simulink model "hdv_hydroelectropowertrain_model"  (R2023b)
settings: Solver=ode1be  StartTime=0.0  StopTime=simulation_length  FixedStep=tsample  MaxStep=tsample
values from neighbouring files (symbols this model uses):
  alpha = 35    [init_model.m]
  Apump = [0 1; 0 0]    [init_model.m]
  available_torque = torque_base+torque_friction_base    [init_model.m]
  Bpump = [0 1]'    [init_model.m]
  btheta_shaft = 2e2    (= 200)    [init_model.m]
  C1 = 10    [init_model.m]
  consumption = [consumption_1, consumption_2, consumption_3, consumption_4,          consumption_5, consumption_6, consumption_7, consumption_8,          consumption_9, consumption_10, consumption_11, consumption_12,          consumption_13, consumption_14, consumption_15, consumption_16          ]    [ic_engine_data.m]
  Cpump = [k 0]    [init_model.m]
  dp_lim = 400    [init_model.m]
  E0 = 3.685    [init_model.m]
  E1 = 0.2156    [init_model.m]
  E2 = 0    [init_model.m]
  E3 = 0    [init_model.m]
  E_1 = -1.031    [init_model.m]
  Elog = -0.05    [init_model.m]
  eta_v_m = 0.98    [init_model.m]
  eta_v_p = 0.97    [init_model.m]
  ki_dp_comp = 1/dp_lim    (= 0.0025)    [init_model.m]
  ki_te_comp = 2/te_lim    [init_model.m]
  kp_ctrl_m = 1    [init_model.m]
  kp_dp_comp = 0.5/dp_lim    (= 0.00125)    [init_model.m]
  kp_te_comp = 1/te_lim    [init_model.m]
  Kpump = acker(Apump,Bpump,poles)    [init_model.m]
  load_blade_enable = 0    [init_model.m]
  Lpump = acker(Apump',Cpump',pole_so)'    [init_model.m]
  M = 125    [init_model.m]
  Ncell = 185    [init_model.m]
  Npump = -1/(Cpump*inv(Apump-Bpump*Kpump)*Bpump)    [init_model.m]
  omega_e_rpm_ref = 1700    [init_model.m]
  omega_l_max_rpm = omega_l_max/(2*pi)*60    (= 50.3075969543)    [init_model.m]
  q1Kalman = tsample^2*1e-2    (= 1e-08)    [init_model.m]
  q2Kalman = tsample^1*1e-1    (= 0.0001)    [init_model.m]
  q3Kalman = 0    [init_model.m]
  Qhr = 400    [init_model.m]
  R0 = 0.015    [init_model.m]
  R1 = 0.015    [init_model.m]
  R_tg = 1.16/2    (= 0.58)    [init_model.m]
  rKalman = 1    [init_model.m]
  rpm_base = [620 700 800 900 1000 1100 1200 1300 1400 1500 1600 1700 1800      1900 2000 2100]    [ic_engine_data.m]
  rpm_consumption = rpm_base    [ic_engine_data.m]
  simulation_length = 245    [init_model.m]
  tau_load = 75e3    (= 75000)    [init_model.m]
  tau_load_max = 1600*41.4    (= 66240)    [init_model.m]
  Tc = tsample    (= 0.001)    [init_model.m]
  torque_base = [max(torque_16_data) max(torque_15_data) max(torque_14_data)      max(torque_13_data) max(torque_12_data) max(torque_11_data)      max(torque_10_data) max(torque_9_data) max(torque_8_data)      max(torque_7_data) max(torque_6_data) max(torque_5_data)      max(torque_4_data) max(torque_3_data) max(torque_2_data)      max(torque_1_data)]    [ic_engine_data.m]
  torque_consumption = torque_reference    [ic_engine_data.m]
  torque_friction_base = -(rpm_base./60*2*pi)*0.25-(rpm_base./60*2*pi).^2*5.2e-4    [ic_engine_data.m]
  tsample = 1e-3    (= 0.001)    [init_model.m]
  v_track1_ref = 8    [init_model.m]
  v_track2_ref = 8    [init_model.m]
  valve_mmorifice_max = 2.75    [init_model.m]
  xv_m_max = 1.2    [init_model.m]
undefined symbols (not defined in the file or in its folder): magnitude
libraries: fl_lib x381, nesl_utility x162, linear_swashplate_ctrl_lib x8, flexshaft_lib x5, bichamber_piston_lib x5, variable_displacement_motor_lib x4, variable_displacement_pump_lib x4, fixed_displacement_pump_lib x4, relief_valve_lib x4, inverse_shuttle_valve_lib x4, hydrostatic_threeway_valve_bichamber_piston_lib x4, hydrostatic_fourway_valve_bichamber_piston_lib x4
(part 8 of 9)

== system hdv_hydroelectropowertrain_model/PR776_powertrain/Hydrostatic_powertrain/driveine_RD1/pressure_charge_system_RD/hydro_check_valve2 ==
  Constant Area Hydraulic Orifice5 : fl_lib/Hydraulic/Hydraulic Elements/Constant Area Hydraulic Orifice  area=1e-4 mm^2  C_d=1  lam_spec=1  B_lam=0.999  Re_cr=12  q_specify=off  q_priority=None  q=0.001 m^3/s  q_nominal_specify=off  q_nominal_unit=m^3/s  q_nominal_value=1  p_specify=off  p_priority=None  p=0 Pa  p_nominal_specify=off  p_nominal_unit=Pa  p_nominal_value=1
      settings: InternalSimscapePortConfiguration="{\"Bottom\":[],\"Left\":[{\"id\":\"A\",\"label\":\"A\",\"type\":\"foundation.hydraulic.hydraulic\"}],\"Right\":[{\"id\":\"B\",\"label\":\"B\",\"type\":\"foundation.hydraulic.hydraulic\"}],\"Top\":[]}"
  Constant Area Hydraulic Orifice6 : fl_lib/Hydraulic/Hydraulic Elements/Constant Area Hydraulic Orifice  area=4 mm^2  C_d=1  lam_spec=1  B_lam=0.999  Re_cr=12  q_specify=off  q_priority=None  q=0.001 m^3/s  q_nominal_specify=off  q_nominal_unit=m^3/s  q_nominal_value=1  p_specify=off  p_priority=None  p=0 Pa  p_nominal_specify=off  p_nominal_unit=Pa  p_nominal_value=1
      settings: InternalSimscapePortConfiguration="{\"Bottom\":[],\"Left\":[{\"id\":\"A\",\"label\":\"A\",\"type\":\"foundation.hydraulic.hydraulic\"}],\"Right\":[{\"id\":\"B\",\"label\":\"B\",\"type\":\"foundation.hydraulic.hydraulic\"}],\"Top\":[]}"
  Hydraulic Flow Rate Sensor : fl_lib/Hydraulic/Hydraulic Sensors/Hydraulic Flow Rate Sensor
  Hydraulic Flow Rate Source : fl_lib/Hydraulic/Hydraulic Sources/Hydraulic Flow Rate Source
      settings: InternalSimscapePortConfiguration="{\"Bottom\":[],\"Left\":[{\"id\":\"P\",\"label\":\"P\",\"type\":\"foundation.hydraulic.hydraulic\"}],\"Right\":[{\"id\":\"S\",\"label\":\"S\",\"type\":\"input\"},{\"id\":\"T\",\"label\":\"T\",\"type\":\"foundation.hydraulic.hydraulic\"}],\"Top\":[]}"
  Hydraulic Pressure Sensor : fl_lib/Hydraulic/Hydraulic Sensors/Hydraulic Pressure Sensor
  Hydraulic Pressure Source2 : fl_lib/Hydraulic/Hydraulic Sources/Hydraulic Pressure Source
      settings: InternalSimscapePortConfiguration="{\"Bottom\":[],\"Left\":[{\"id\":\"P\",\"label\":\"P\",\"type\":\"foundation.hydraulic.hydraulic\"}],\"Right\":[{\"id\":\"S\",\"label\":\"S\",\"type\":\"input\"},{\"id\":\"T\",\"label\":\"T\",\"type\":\"foundation.hydraulic.hydraulic\"}],\"Top\":[]}"
  Hydraulic Reference : fl_lib/Hydraulic/Hydraulic Elements/Hydraulic Reference
  PS Saturation : fl_lib/Physical Signals/Nonlinear Operators/PS Saturation  upper_limit=inf m^3/s  lower_limit=0 m^3/s
  PS Saturation1 : fl_lib/Physical Signals/Nonlinear Operators/PS Saturation  upper_limit=inf Pa  lower_limit=0 Pa
  PS Transfer Function : fl_lib/Physical Signals/Linear Operators/PS Transfer Function  transfer_function_type=foundation.enum.transfer_function_type.lag  T=tsample s  T1=2 s  T2=1 s  reset_method=foundation.enum.IntegratorResetSpec.None  initial_condition_spec=foundation.enum.IntegratorICSpec.Internal  y0=0 m^3/s
      settings: InternalSimscapePortConfiguration="{\"Bottom\":[],\"Left\":[{\"id\":\"U\",\"label\":\"\",\"type\":\"input\"}],\"Right\":[{\"id\":\"Y\",\"label\":\"\",\"type\":\"output\"}],\"Top\":[]}"
  PS Transfer Function1 : fl_lib/Physical Signals/Linear Operators/PS Transfer Function  transfer_function_type=foundation.enum.transfer_function_type.lag  T=tsample s  T1=2 s  T2=1 s  reset_method=foundation.enum.IntegratorResetSpec.None  initial_condition_spec=foundation.enum.IntegratorICSpec.Internal  y0=0 Pa
      settings: InternalSimscapePortConfiguration="{\"Bottom\":[],\"Left\":[{\"id\":\"U\",\"label\":\"\",\"type\":\"input\"}],\"Right\":[{\"id\":\"Y\",\"label\":\"\",\"type\":\"output\"}],\"Top\":[]}"
  A : PMIOPort  Side=Left
  B : PMIOPort  Port=2  Side=Right
  connections:
  PS Transfer Function/LConn1 -- PS Saturation/RConn1
  PS Saturation1/RConn1 -- PS Transfer Function1/LConn1
  PS Transfer Function/RConn1 -- Hydraulic Flow Rate Source/RConn1
  Constant Area Hydraulic Orifice5/LConn1 -- A/RConn1 -- Hydraulic Pressure Sensor/LConn1 -- Hydraulic Flow Rate Source/RConn2
  Hydraulic Pressure Sensor/RConn2 -- PS Saturation1/LConn1
  PS Transfer Function1/RConn1 -- Hydraulic Pressure Source2/RConn1
  PS Saturation/LConn1 -- Hydraulic Flow Rate Sensor/RConn1
  B/RConn1 -- Constant Area Hydraulic Orifice5/RConn1 -- Hydraulic Pressure Sensor/RConn1 -- Hydraulic Flow Rate Source/LConn1
  Hydraulic Pressure Source2/LConn1 -- Hydraulic Flow Rate Sensor/LConn1
  Hydraulic Pressure Source2/RConn2 -- Hydraulic Reference/LConn1 -- Constant Area Hydraulic Orifice6/RConn1
  Hydraulic Flow Rate Sensor/RConn2 -- Constant Area Hydraulic Orifice6/LConn1

== system hdv_hydroelectropowertrain_model/PR776_powertrain/Hydrostatic_powertrain/driveine_RD1/vd_ctrl_motor_RD/hose3 ==
  Constant Area Hydraulic Orifice : fl_lib/Hydraulic/Hydraulic Elements/Constant Area Hydraulic Orifice  area=1e-8 m^2  C_d=0.7  lam_spec=1  B_lam=0.999  Re_cr=12  q_specify=off  q_priority=None  q=0.001 m^3/s  q_nominal_specify=off  q_nominal_unit=m^3/s  q_nominal_value=1  p_specify=off  p_priority=None  p=0 Pa  p_nominal_specify=off  p_nominal_unit=Pa  p_nominal_value=1
      settings: InternalSimscapePortConfiguration="{\"Bottom\":[],\"Left\":[{\"id\":\"A\",\"label\":\"A\",\"type\":\"foundation.hydraulic.hydraulic\"}],\"Right\":[{\"id\":\"B\",\"label\":\"B\",\"type\":\"foundation.hydraulic.hydraulic\"}],\"Top\":[]}"
  Constant Area Hydraulic Orifice1 : fl_lib/Hydraulic/Hydraulic Elements/Constant Area Hydraulic Orifice  area=1e-8 m^2  C_d=0.7  lam_spec=1  B_lam=0.999  Re_cr=12  q_specify=off  q_priority=None  q=0.001 m^3/s  q_nominal_specify=off  q_nominal_unit=m^3/s  q_nominal_value=1  p_specify=off  p_priority=None  p=0 Pa  p_nominal_specify=off  p_nominal_unit=Pa  p_nominal_value=1
      settings: InternalSimscapePortConfiguration="{\"Bottom\":[],\"Left\":[{\"id\":\"A\",\"label\":\"A\",\"type\":\"foundation.hydraulic.hydraulic\"}],\"Right\":[{\"id\":\"B\",\"label\":\"B\",\"type\":\"foundation.hydraulic.hydraulic\"}],\"Top\":[]}"
  Hydraulic Flow Rate Sensor3 : fl_lib/Hydraulic/Hydraulic Sensors/Hydraulic Flow Rate Sensor
  Hydraulic Flow Rate Source : fl_lib/Hydraulic/Hydraulic Sources/Hydraulic Flow Rate Source
      settings: InternalSimscapePortConfiguration="{\"Bottom\":[],\"Left\":[{\"id\":\"P\",\"label\":\"P\",\"type\":\"foundation.hydraulic.hydraulic\"}],\"Right\":[{\"id\":\"S\",\"label\":\"S\",\"type\":\"input\"},{\"id\":\"T\",\"label\":\"T\",\"type\":\"foundation.hydraulic.hydraulic\"}],\"Top\":[]}"
  Hydraulic Pressure Sensor2 : fl_lib/Hydraulic/Hydraulic Sensors/Hydraulic Pressure Sensor
  Hydraulic Pressure Source : fl_lib/Hydraulic/Hydraulic Sources/Hydraulic Pressure Source
      settings: InternalSimscapePortConfiguration="{\"Bottom\":[],\"Left\":[{\"id\":\"P\",\"label\":\"P\",\"type\":\"foundation.hydraulic.hydraulic\"}],\"Right\":[{\"id\":\"S\",\"label\":\"S\",\"type\":\"input\"},{\"id\":\"T\",\"label\":\"T\",\"type\":\"foundation.hydraulic.hydraulic\"}],\"Top\":[]}"
  Hydraulic Reference : fl_lib/Hydraulic/Hydraulic Elements/Hydraulic Reference
  PS Gain : fl_lib/Physical Signals/Functions/PS Gain  gain=1 Pa
  PS Gain1 : fl_lib/Physical Signals/Functions/PS Gain  gain=1 Pa^-1
  PS Gain2 : fl_lib/Physical Signals/Functions/PS Gain  gain=1 m^3/s
  PS Gain3 : fl_lib/Physical Signals/Functions/PS Gain  gain=1 m^-3*s
  PS Transfer Function : fl_lib/Physical Signals/Linear Operators/PS Transfer Function  transfer_function_type=foundation.enum.transfer_function_type.lag  T=0.01 s  T1=2 s  T2=1 s  reset_method=foundation.enum.IntegratorResetSpec.None  initial_condition_spec=foundation.enum.IntegratorICSpec.Internal  y0=0
      settings: InternalSimscapePortConfiguration="{\"Bottom\":[],\"Left\":[{\"id\":\"U\",\"label\":\"\",\"type\":\"input\"}],\"Right\":[{\"id\":\"Y\",\"label\":\"\",\"type\":\"output\"}],\"Top\":[]}"
  PS Transfer Function1 : fl_lib/Physical Signals/Linear Operators/PS Transfer Function  transfer_function_type=foundation.enum.transfer_function_type.lag  T=0.01 s  T1=2 s  T2=1 s  reset_method=foundation.enum.IntegratorResetSpec.None  initial_condition_spec=foundation.enum.IntegratorICSpec.Internal  y0=0
      settings: InternalSimscapePortConfiguration="{\"Bottom\":[],\"Left\":[{\"id\":\"U\",\"label\":\"\",\"type\":\"input\"}],\"Right\":[{\"id\":\"Y\",\"label\":\"\",\"type\":\"output\"}],\"Top\":[]}"
  A : PMIOPort  Side=Left
  AA : PMIOPort  Port=2  Side=Right
  B : PMIOPort  Port=3  Side=Left
  BB : PMIOPort  Port=4  Side=Right
  connections:
  AA/RConn1 -- Constant Area Hydraulic Orifice1/LConn1 -- Hydraulic Flow Rate Sensor3/RConn2
  PS Gain2/RConn1 -- Hydraulic Flow Rate Source/RConn1
  Hydraulic Flow Rate Sensor3/RConn1 -- PS Gain3/LConn1
  Hydraulic Flow Rate Sensor3/LConn1 -- Hydraulic Pressure Source/LConn1
  Hydraulic Pressure Source/RConn1 -- PS Gain/RConn1
  PS Gain1/LConn1 -- Hydraulic Pressure Sensor2/RConn2
  Hydraulic Pressure Source/RConn2 -- Hydraulic Pressure Sensor2/RConn1 -- Constant Area Hydraulic Orifice/RConn1 -- B/RConn1 -- Hydraulic Flow Rate Source/LConn1 -- Constant Area Hydraulic Orifice1/RConn1 -- Hydraulic Reference/LConn1 -- BB/RConn1
  PS Transfer Function1/RConn1 -- PS Gain2/LConn1
  PS Transfer Function/RConn1 -- PS Gain/LConn1
  A/RConn1 -- Constant Area Hydraulic Orifice/LConn1 -- Hydraulic Pressure Sensor2/LConn1 -- Hydraulic Flow Rate Source/RConn2
  PS Gain3/RConn1 -- PS Transfer Function1/LConn1
  PS Gain1/RConn1 -- PS Transfer Function/LConn1

== system hdv_hydroelectropowertrain_model/PR776_powertrain/Hydrostatic_powertrain/driveine_RD1/vd_ctrl_motor_RD/servo motor LD ==
  displacement reference pu : Inport
  PS Add : fl_lib/Physical Signals/Functions/PS Add
  PS Constant : fl_lib/Physical Signals/Sources/PS Constant  constant=1
  PS Gain : fl_lib/Physical Signals/Functions/PS Gain  gain=-1/0.06 m^-1
  hydrostatic_threeway_valve_bichamber_piston : hydrostatic_threeway_valve_bichamber_piston_lib/hydrostatic_threeway_valve_bichamber_piston  Dh=Dh m  Dr=Dr m  Lp=Lpm m  xv_max=xv_m_max mm  mp=mp_m kg  kp=kp_m N/m  bp=bp_m N/(m/s)  qs_specify=off  qs_priority=None  qs=0 m^3/s  qs_nominal_specify=off  qs_nominal_unit=m^3/s  qs_nominal_value=1  qv_specify=off  qv_priority=None  qv=0 m^3/s  qv_nominal_specify=off  qv_nominal_unit=m^3/s  qv_nominal_value=1  q_specify=off  q_priority=None  q=0 m^3/s  q_nominal_specify=off  q_nominal_unit=m^3/s  q_nominal_value=1  q_leak_specify=off  q_leak_priority=None  q_leak=0 m^3/s  q_leak_nominal_specify=off  q_leak_nominal_unit=m^3/s  q_leak_nominal_value=1  pc_specify=off  pc_priority=None  pc=0 bar  pc_nominal_specify=off  pc_nominal_unit=bar  pc_nominal_value=1  fp_specify=off  fp_priority=None  fp=0 N  fp_nominal_specify=off  fp_nominal_unit=N  fp_nominal_value=1  vp_specify=off  vp_priority=None  vp=0 m/s  vp_nominal_specify=off  vp_nominal_unit=m/s  vp_nominal_value=1  xp_specify=off  xp_priority=High  xp=10 mm  xp_nominal_specify=off  xp_nominal_unit=mm  xp_nominal_value=1
      settings: InternalSimscapePortConfiguration="{\"Bottom\":[],\"Left\":[{\"id\":\"xv\",\"label\":\"xv\",\"type\":\"input\"},{\"id\":\"cA\",\"label\":\"cA\",\"type\":\"foundation.hydraulic.hydraulic\"},{\"id\":\"cB\",\"label\":\"cB\",\"type\":\"foundation.hydraulic.hydraulic\"}],\"Right\":[{\"id\":\"P\",\"label\":\"P\",\"type\":\"foundation.mechanical.translational.translational\"},{\"id\":\"xp_out\",\"label\":\"xp\",\"type\":\"output\"},{\"id\":\"mforce\",\"label\":\"fm\",\"type\":\"output\"},{\"id\":\"flowC\",\"label\":\"flowC\",\"type\":\"output\"},{\"id\":\"pC\",\"label\":\"pC\",\"type\":\"output\"}],\"Top\":[]}"
  servo_ctrl : Subsystem
  pS : PMIOPort  Side=Left
  pT : PMIOPort  Port=2  Side=Left
  vd : PMIOPort  Port=3  Side=Right
  wires:
  displacement reference pu/1 -> servo_ctrl/1(ref)
  connections:
  hydrostatic_threeway_valve_bichamber_piston/LConn3 -- pT/RConn1
  hydrostatic_threeway_valve_bichamber_piston/LConn2 -- pS/RConn1
  hydrostatic_threeway_valve_bichamber_piston/RConn2 -- PS Gain/LConn1 -- servo_ctrl/LConn1
  hydrostatic_threeway_valve_bichamber_piston/LConn1 -- servo_ctrl/RConn1
  vd/RConn1 -- PS Add/RConn1
  PS Gain/RConn1 -- PS Add/LConn1
  PS Constant/RConn1 -- PS Add/LConn2

== system hdv_hydroelectropowertrain_model/PR776_powertrain/Hydrostatic_powertrain/driveine_RD1/vd_ctrl_pump_RD/hose3 ==
  Constant Area Hydraulic Orifice : fl_lib/Hydraulic/Hydraulic Elements/Constant Area Hydraulic Orifice  area=1e-8 m^2  C_d=0.7  lam_spec=1  B_lam=0.999  Re_cr=12  q_specify=off  q_priority=None  q=0.001 m^3/s  q_nominal_specify=off  q_nominal_unit=m^3/s  q_nominal_value=1  p_specify=off  p_priority=None  p=0 Pa  p_nominal_specify=off  p_nominal_unit=Pa  p_nominal_value=1
      settings: InternalSimscapePortConfiguration="{\"Bottom\":[],\"Left\":[{\"id\":\"A\",\"label\":\"A\",\"type\":\"foundation.hydraulic.hydraulic\"}],\"Right\":[{\"id\":\"B\",\"label\":\"B\",\"type\":\"foundation.hydraulic.hydraulic\"}],\"Top\":[]}"
  Constant Area Hydraulic Orifice1 : fl_lib/Hydraulic/Hydraulic Elements/Constant Area Hydraulic Orifice  area=1e-8 m^2  C_d=0.7  lam_spec=1  B_lam=0.999  Re_cr=12  q_specify=off  q_priority=None  q=0.001 m^3/s  q_nominal_specify=off  q_nominal_unit=m^3/s  q_nominal_value=1  p_specify=off  p_priority=None  p=0 Pa  p_nominal_specify=off  p_nominal_unit=Pa  p_nominal_value=1
      settings: InternalSimscapePortConfiguration="{\"Bottom\":[],\"Left\":[{\"id\":\"A\",\"label\":\"A\",\"type\":\"foundation.hydraulic.hydraulic\"}],\"Right\":[{\"id\":\"B\",\"label\":\"B\",\"type\":\"foundation.hydraulic.hydraulic\"}],\"Top\":[]}"
  Hydraulic Flow Rate Sensor3 : fl_lib/Hydraulic/Hydraulic Sensors/Hydraulic Flow Rate Sensor
  Hydraulic Flow Rate Source : fl_lib/Hydraulic/Hydraulic Sources/Hydraulic Flow Rate Source
      settings: InternalSimscapePortConfiguration="{\"Bottom\":[],\"Left\":[{\"id\":\"P\",\"label\":\"P\",\"type\":\"foundation.hydraulic.hydraulic\"}],\"Right\":[{\"id\":\"S\",\"label\":\"S\",\"type\":\"input\"},{\"id\":\"T\",\"label\":\"T\",\"type\":\"foundation.hydraulic.hydraulic\"}],\"Top\":[]}"
  Hydraulic Pressure Sensor2 : fl_lib/Hydraulic/Hydraulic Sensors/Hydraulic Pressure Sensor
  Hydraulic Pressure Source : fl_lib/Hydraulic/Hydraulic Sources/Hydraulic Pressure Source
      settings: InternalSimscapePortConfiguration="{\"Bottom\":[],\"Left\":[{\"id\":\"P\",\"label\":\"P\",\"type\":\"foundation.hydraulic.hydraulic\"}],\"Right\":[{\"id\":\"S\",\"label\":\"S\",\"type\":\"input\"},{\"id\":\"T\",\"label\":\"T\",\"type\":\"foundation.hydraulic.hydraulic\"}],\"Top\":[]}"
  Hydraulic Reference : fl_lib/Hydraulic/Hydraulic Elements/Hydraulic Reference
  PS Gain : fl_lib/Physical Signals/Functions/PS Gain  gain=1 Pa
  PS Gain1 : fl_lib/Physical Signals/Functions/PS Gain  gain=1 Pa^-1
  PS Gain2 : fl_lib/Physical Signals/Functions/PS Gain  gain=1 m^3/s
  PS Gain3 : fl_lib/Physical Signals/Functions/PS Gain  gain=1 m^-3*s
  PS Transfer Function : fl_lib/Physical Signals/Linear Operators/PS Transfer Function  transfer_function_type=foundation.enum.transfer_function_type.lag  T=0.01 s  T1=2 s  T2=1 s  reset_method=foundation.enum.IntegratorResetSpec.None  initial_condition_spec=foundation.enum.IntegratorICSpec.Internal  y0=0
      settings: InternalSimscapePortConfiguration="{\"Bottom\":[],\"Left\":[{\"id\":\"U\",\"label\":\"\",\"type\":\"input\"}],\"Right\":[{\"id\":\"Y\",\"label\":\"\",\"type\":\"output\"}],\"Top\":[]}"
  PS Transfer Function1 : fl_lib/Physical Signals/Linear Operators/PS Transfer Function  transfer_function_type=foundation.enum.transfer_function_type.lag  T=0.01 s  T1=2 s  T2=1 s  reset_method=foundation.enum.IntegratorResetSpec.None  initial_condition_spec=foundation.enum.IntegratorICSpec.Internal  y0=0
      settings: InternalSimscapePortConfiguration="{\"Bottom\":[],\"Left\":[{\"id\":\"U\",\"label\":\"\",\"type\":\"input\"}],\"Right\":[{\"id\":\"Y\",\"label\":\"\",\"type\":\"output\"}],\"Top\":[]}"
  A : PMIOPort  Side=Left
  AA : PMIOPort  Port=2  Side=Right
  B : PMIOPort  Port=3  Side=Left
  BB : PMIOPort  Port=4  Side=Right
  connections:
  AA/RConn1 -- Constant Area Hydraulic Orifice1/LConn1 -- Hydraulic Flow Rate Sensor3/RConn2
  PS Gain2/RConn1 -- Hydraulic Flow Rate Source/RConn1
  Hydraulic Flow Rate Sensor3/RConn1 -- PS Gain3/LConn1
  Hydraulic Flow Rate Sensor3/LConn1 -- Hydraulic Pressure Source/LConn1
  Hydraulic Pressure Source/RConn1 -- PS Gain/RConn1
  PS Gain1/LConn1 -- Hydraulic Pressure Sensor2/RConn2
  Hydraulic Pressure Source/RConn2 -- Hydraulic Pressure Sensor2/RConn1 -- Constant Area Hydraulic Orifice/RConn1 -- B/RConn1 -- Hydraulic Flow Rate Source/LConn1 -- Constant Area Hydraulic Orifice1/RConn1 -- Hydraulic Reference/LConn1 -- BB/RConn1
  PS Transfer Function1/RConn1 -- PS Gain2/LConn1
  PS Transfer Function/RConn1 -- PS Gain/LConn1
  A/RConn1 -- Constant Area Hydraulic Orifice/LConn1 -- Hydraulic Pressure Sensor2/LConn1 -- Hydraulic Flow Rate Source/RConn2
  PS Gain3/RConn1 -- PS Transfer Function1/LConn1
  PS Gain1/RConn1 -- PS Transfer Function/LConn1

== system hdv_hydroelectropowertrain_model/PR776_powertrain/Hydrostatic_powertrain/driveine_RD1/vd_ctrl_pump_RD/servo pump RD ==
  displacement reference pu : Inport
  Gain : Gain  Gain=0.03647/2
  PS Gain : fl_lib/Physical Signals/Functions/PS Gain  gain=1/(0.03647/2) m^-1
  PS-Simulink Converter7 : nesl_utility/PS-Simulink Converter  PhysicalDomain=network_engine_domain  SubClassName=ps_output  LeftPortType=input  RightPortType=output  PseudoPeriodic=off  Frequencies=[]  VectorFormat=1-D array  Unit=1  AffineConversion=off
  hydrostatic_fourway_valve_bichamber : hydrostatic_fourway_valve_bichamber_piston_lib/hydrostatic_fourway_valve_bichamber  D1=D1 m  D2=D2 m  Lp=Lp m  xv_max=xv_max mm  mp=mp kg  kp=kp N/m  bp=bp N/(m/s)  q1_specify=off  q1_priority=None  q1=0 m^3/s  q1_nominal_specify=off  q1_nominal_unit=m^3/s  q1_nominal_value=1  q2_specify=off  q2_priority=None  q2=0 m^3/s  q2_nominal_specify=off  q2_nominal_unit=m^3/s  q2_nominal_value=1  qin_specify=off  qin_priority=None  qin=0 m^3/s  qin_nominal_specify=off  qin_nominal_unit=m^3/s  qin_nominal_value=1  qout_specify=off  qout_priority=None  qout=0 m^3/s  qout_nominal_specify=off  qout_nominal_unit=m^3/s  qout_nominal_value=1  p1_specify=off  p1_priority=High  p1=125 bar  p1_nominal_specify=off  p1_nominal_unit=bar  p1_nominal_value=1  p2_specify=off  p2_priority=High  p2=125 bar  p2_nominal_specify=off  p2_nominal_unit=bar  p2_nominal_value=1  fp_specify=off  fp_priority=None  fp=0 N  fp_nominal_specify=off  fp_nominal_unit=N  fp_nominal_value=1  vp_specify=off  vp_priority=None  vp=0 m/s  vp_nominal_specify=off  vp_nominal_unit=m/s  vp_nominal_value=1  xp_specify=off  xp_priority=High  xp=500 mm  xp_nominal_specify=off  xp_nominal_unit=mm  xp_nominal_value=1
      settings: InternalSimscapePortConfiguration="{\"Bottom\":[],\"Left\":[{\"id\":\"xv\",\"label\":\"xv\",\"type\":\"input\"},{\"id\":\"S\",\"label\":\"S\",\"type\":\"foundation.hydraulic.hydraulic\"},{\"id\":\"T\",\"label\":\"T\",\"type\":\"foundation.hydraulic.hydraulic\"}],\"Right\":[{\"id\":\"P\",\"label\":\"P\",\"type\":\"foundation.mechanical.translational.translational\"},{\"id\":\"xp_out\",\"label\":\"xp\",\"type\":\"output\"},{\"id\":\"q1_out\",\"label\":\"q1\",\"type\":\"output\"},{\"id\":\"q2_out\",\"label\":\"q2\",\"type\":\"output\"},{\"id\":\"p1_out\",\"label\":\"p1\",\"type\":\"output\"},{\"id\":\"p2_out\",\"label\":\"p2\",\"type\":\"output\"}],\"Top\":[]}"
  pmlinear_actuator : pm_linear_actuator_lib/pmlinear_actuator  Bm=1 s*V/m^2  mv=mv kg  Lc=Lc H  Rc=Rc Ohm  bv=bv N/(m/s)  h=h m  xv_max=xv_max mm  n=n  ic_specify=off  ic_priority=High  ic=0 A  ic_nominal_specify=off  ic_nominal_unit=A  ic_nominal_value=1  vv_specify=off  vv_priority=None  vv=0 m/s  vv_nominal_specify=off  vv_nominal_unit=m/s  vv_nominal_value=1  xv_specify=off  xv_priority=None  xv=0 m  xv_nominal_specify=off  xv_nominal_unit=m  xv_nominal_value=1
      settings: InternalSimscapePortConfiguration="{\"Bottom\":[],\"Left\":[{\"id\":\"uc\",\"label\":\"uc\",\"type\":\"input\"}],\"Right\":[{\"id\":\"xv_out\",\"label\":\"xv\",\"type\":\"output\"}],\"Top\":[]}"
  servo_ctrl : Subsystem
  pS : PMIOPort  Side=Left
  pT : PMIOPort  Port=2  Side=Left
  vd pu : PMIOPort  Port=3  Side=Right
  wires:
  Gain/1 -> servo_ctrl/1(ref)
  PS-Simulink Converter7/1 -> servo_ctrl/2(xp)  "xp"
  displacement reference pu/1 -> Gain/1
  connections:
  hydrostatic_fourway_valve_bichamber/LConn3 -- pT/RConn1
  hydrostatic_fourway_valve_bichamber/LConn2 -- pS/RConn1
  hydrostatic_fourway_valve_bichamber/RConn2 -- PS Gain/LConn1 -- PS-Simulink Converter7/LConn1
  servo_ctrl/RConn1 -- pmlinear_actuator/LConn1
  pmlinear_actuator/RConn1 -- hydrostatic_fourway_valve_bichamber/LConn1
  PS Gain/RConn1 -- vd pu/RConn1

== system hdv_hydroelectropowertrain_model/PR776_powertrain/Hydrostatic_powertrain/driveline_RD2/pressure_charge_system_RD/Subsystem ==
  Fixed displacement pump : fixed_displacement_pump_lib/Fixed displacement pump  max_Dv=27 cm^3/rev  inertia_pump=0.05 kg*m^2  oil_vol=2.0 l  bp=0.0025 N*m/(rad/s)  lk=1e-6 m  t_specify=off  t_priority=None  t=0 N*m  t_nominal_specify=off  t_nominal_unit=N*m  t_nominal_value=1  q_specify=off  q_priority=None  q=0 m^3/s  q_nominal_specify=off  q_nominal_unit=m^3/s  q_nominal_value=1  qt_specify=off  qt_priority=None  qt=0 m^3/s  qt_nominal_specify=off  qt_nominal_unit=m^3/s  qt_nominal_value=1  qleak_specify=off  qleak_priority=None  qleak=0 m^3/s  qleak_nominal_specify=off  qleak_nominal_unit=m^3/s  qleak_nominal_value=1  Dv_specify=off  Dv_priority=None  Dv=0 cm^3  Dv_nominal_specify=off  Dv_nominal_unit=cm^3  Dv_nominal_value=1  dp_specify=off  dp_priority=None  dp=0 Pa  dp_nominal_specify=off  dp_nominal_unit=Pa  dp_nominal_value=1  we_specify=off  we_priority=None  we=0 rad/s  we_nominal_specify=off  we_nominal_unit=rad/s  we_nominal_value=1
      settings: InternalSimscapePortConfiguration="{\"Bottom\":[],\"Left\":[{\"id\":\"C\",\"label\":\"C\",\"type\":\"foundation.mechanical.rotational.rotational\"}],\"Right\":[{\"id\":\"A\",\"label\":\"A\",\"type\":\"foundation.hydraulic.hydraulic\"},{\"id\":\"B\",\"label\":\"B\",\"type\":\"foundation.hydraulic.hydraulic\"}],\"Top\":[]}"
  Hydraulic Reference3 : fl_lib/Hydraulic/Hydraulic Elements/Hydraulic Reference
  Hydraulic Reference4 : fl_lib/Hydraulic/Hydraulic Elements/Hydraulic Reference
  relief valve : relief_valve_lib/relief valve  dp_ref=32 bar  pnom=32 bar  p_set=32 bar  p_reg=12 bar  x_rv_max=12.0 mm  qA_specify=off  qA_priority=None  qA=0 m^3/s  qA_nominal_specify=off  qA_nominal_unit=m^3/s  qA_nominal_value=1  qB_specify=off  qB_priority=None  qB=0 m^3/s  qB_nominal_specify=off  qB_nominal_unit=m^3/s  qB_nominal_value=1  dp_specify=off  dp_priority=None  dp=0 Pa  dp_nominal_specify=off  dp_nominal_unit=Pa  dp_nominal_value=1  x_rv_specify=off  x_rv_priority=None  x_rv=0 m  x_rv_nominal_specify=off  x_rv_nominal_unit=m  x_rv_nominal_value=1  x_rv_flt_specify=off  x_rv_flt_priority=None  x_rv_flt=0 m  x_rv_flt_nominal_specify=off  x_rv_flt_nominal_unit=m  x_rv_flt_nominal_value=1
      settings: LogSimulationData=on  InternalSimscapePortConfiguration="{\"Bottom\":[],\"Left\":[{\"id\":\"cA\",\"label\":\"cA\",\"type\":\"foundation.hydraulic.hydraulic\"}],\"Right\":[{\"id\":\"cB\",\"label\":\"cB\",\"type\":\"foundation.hydraulic.hydraulic\"}],\"Top\":[]}"
  ps : PMIOPort  Side=Right
  D : PMIOPort  Port=2  Side=Left
  connections:
  Fixed displacement pump/LConn1 -- D/RConn1
  Fixed displacement pump/RConn2 -- Hydraulic Reference3/LConn1
  Hydraulic Reference4/LConn1 -- relief valve/RConn1
  relief valve/LConn1 -- ps/RConn1 -- Fixed displacement pump/RConn1

== system hdv_hydroelectropowertrain_model/PR776_powertrain/Hydrostatic_powertrain/driveline_RD2/pressure_charge_system_RD/hydro_check_valve1 ==
  Constant Area Hydraulic Orifice5 : fl_lib/Hydraulic/Hydraulic Elements/Constant Area Hydraulic Orifice  area=1e-4 mm^2  C_d=1  lam_spec=1  B_lam=0.999  Re_cr=12  q_specify=off  q_priority=None  q=0.001 m^3/s  q_nominal_specify=off  q_nominal_unit=m^3/s  q_nominal_value=1  p_specify=off  p_priority=None  p=0 Pa  p_nominal_specify=off  p_nominal_unit=Pa  p_nominal_value=1
      settings: InternalSimscapePortConfiguration="{\"Bottom\":[],\"Left\":[{\"id\":\"A\",\"label\":\"A\",\"type\":\"foundation.hydraulic.hydraulic\"}],\"Right\":[{\"id\":\"B\",\"label\":\"B\",\"type\":\"foundation.hydraulic.hydraulic\"}],\"Top\":[]}"
  Constant Area Hydraulic Orifice6 : fl_lib/Hydraulic/Hydraulic Elements/Constant Area Hydraulic Orifice  area=4 mm^2  C_d=1  lam_spec=1  B_lam=0.999  Re_cr=12  q_specify=off  q_priority=None  q=0.001 m^3/s  q_nominal_specify=off  q_nominal_unit=m^3/s  q_nominal_value=1  p_specify=off  p_priority=None  p=0 Pa  p_nominal_specify=off  p_nominal_unit=Pa  p_nominal_value=1
      settings: InternalSimscapePortConfiguration="{\"Bottom\":[],\"Left\":[{\"id\":\"A\",\"label\":\"A\",\"type\":\"foundation.hydraulic.hydraulic\"}],\"Right\":[{\"id\":\"B\",\"label\":\"B\",\"type\":\"foundation.hydraulic.hydraulic\"}],\"Top\":[]}"
  Hydraulic Flow Rate Sensor : fl_lib/Hydraulic/Hydraulic Sensors/Hydraulic Flow Rate Sensor
  Hydraulic Flow Rate Source : fl_lib/Hydraulic/Hydraulic Sources/Hydraulic Flow Rate Source
      settings: InternalSimscapePortConfiguration="{\"Bottom\":[],\"Left\":[{\"id\":\"P\",\"label\":\"P\",\"type\":\"foundation.hydraulic.hydraulic\"}],\"Right\":[{\"id\":\"S\",\"label\":\"S\",\"type\":\"input\"},{\"id\":\"T\",\"label\":\"T\",\"type\":\"foundation.hydraulic.hydraulic\"}],\"Top\":[]}"
  Hydraulic Pressure Sensor : fl_lib/Hydraulic/Hydraulic Sensors/Hydraulic Pressure Sensor
  Hydraulic Pressure Source2 : fl_lib/Hydraulic/Hydraulic Sources/Hydraulic Pressure Source
      settings: InternalSimscapePortConfiguration="{\"Bottom\":[],\"Left\":[{\"id\":\"P\",\"label\":\"P\",\"type\":\"foundation.hydraulic.hydraulic\"}],\"Right\":[{\"id\":\"S\",\"label\":\"S\",\"type\":\"input\"},{\"id\":\"T\",\"label\":\"T\",\"type\":\"foundation.hydraulic.hydraulic\"}],\"Top\":[]}"
  Hydraulic Reference : fl_lib/Hydraulic/Hydraulic Elements/Hydraulic Reference
  PS Saturation : fl_lib/Physical Signals/Nonlinear Operators/PS Saturation  upper_limit=inf m^3/s  lower_limit=0 m^3/s
  PS Saturation1 : fl_lib/Physical Signals/Nonlinear Operators/PS Saturation  upper_limit=inf Pa  lower_limit=0 Pa
  PS Transfer Function : fl_lib/Physical Signals/Linear Operators/PS Transfer Function  transfer_function_type=foundation.enum.transfer_function_type.lag  T=tsample s  T1=2 s  T2=1 s  reset_method=foundation.enum.IntegratorResetSpec.None  initial_condition_spec=foundation.enum.IntegratorICSpec.Internal  y0=0 m^3/s
      settings: InternalSimscapePortConfiguration="{\"Bottom\":[],\"Left\":[{\"id\":\"U\",\"label\":\"\",\"type\":\"input\"}],\"Right\":[{\"id\":\"Y\",\"label\":\"\",\"type\":\"output\"}],\"Top\":[]}"
  PS Transfer Function1 : fl_lib/Physical Signals/Linear Operators/PS Transfer Function  transfer_function_type=foundation.enum.transfer_function_type.lag  T=tsample s  T1=2 s  T2=1 s  reset_method=foundation.enum.IntegratorResetSpec.None  initial_condition_spec=foundation.enum.IntegratorICSpec.Internal  y0=0 Pa
      settings: InternalSimscapePortConfiguration="{\"Bottom\":[],\"Left\":[{\"id\":\"U\",\"label\":\"\",\"type\":\"input\"}],\"Right\":[{\"id\":\"Y\",\"label\":\"\",\"type\":\"output\"}],\"Top\":[]}"
  A : PMIOPort  Side=Left
  B : PMIOPort  Port=2  Side=Right
  connections:
  PS Transfer Function/LConn1 -- PS Saturation/RConn1
  PS Saturation1/RConn1 -- PS Transfer Function1/LConn1
  PS Transfer Function/RConn1 -- Hydraulic Flow Rate Source/RConn1
  Constant Area Hydraulic Orifice5/LConn1 -- A/RConn1 -- Hydraulic Pressure Sensor/LConn1 -- Hydraulic Flow Rate Source/RConn2
  Hydraulic Pressure Sensor/RConn2 -- PS Saturation1/LConn1
  PS Transfer Function1/RConn1 -- Hydraulic Pressure Source2/RConn1
  PS Saturation/LConn1 -- Hydraulic Flow Rate Sensor/RConn1
  B/RConn1 -- Constant Area Hydraulic Orifice5/RConn1 -- Hydraulic Pressure Sensor/RConn1 -- Hydraulic Flow Rate Source/LConn1
  Hydraulic Pressure Source2/LConn1 -- Hydraulic Flow Rate Sensor/LConn1
  Hydraulic Pressure Source2/RConn2 -- Hydraulic Reference/LConn1 -- Constant Area Hydraulic Orifice6/RConn1
  Hydraulic Flow Rate Sensor/RConn2 -- Constant Area Hydraulic Orifice6/LConn1

== system hdv_hydroelectropowertrain_model/PR776_powertrain/Hydrostatic_powertrain/driveline_RD2/pressure_charge_system_RD/hydro_check_valve2 ==
  Constant Area Hydraulic Orifice5 : fl_lib/Hydraulic/Hydraulic Elements/Constant Area Hydraulic Orifice  area=1e-4 mm^2  C_d=1  lam_spec=1  B_lam=0.999  Re_cr=12  q_specify=off  q_priority=None  q=0.001 m^3/s  q_nominal_specify=off  q_nominal_unit=m^3/s  q_nominal_value=1  p_specify=off  p_priority=None  p=0 Pa  p_nominal_specify=off  p_nominal_unit=Pa  p_nominal_value=1
      settings: InternalSimscapePortConfiguration="{\"Bottom\":[],\"Left\":[{\"id\":\"A\",\"label\":\"A\",\"type\":\"foundation.hydraulic.hydraulic\"}],\"Right\":[{\"id\":\"B\",\"label\":\"B\",\"type\":\"foundation.hydraulic.hydraulic\"}],\"Top\":[]}"
  Constant Area Hydraulic Orifice6 : fl_lib/Hydraulic/Hydraulic Elements/Constant Area Hydraulic Orifice  area=4 mm^2  C_d=1  lam_spec=1  B_lam=0.999  Re_cr=12  q_specify=off  q_priority=None  q=0.001 m^3/s  q_nominal_specify=off  q_nominal_unit=m^3/s  q_nominal_value=1  p_specify=off  p_priority=None  p=0 Pa  p_nominal_specify=off  p_nominal_unit=Pa  p_nominal_value=1
      settings: InternalSimscapePortConfiguration="{\"Bottom\":[],\"Left\":[{\"id\":\"A\",\"label\":\"A\",\"type\":\"foundation.hydraulic.hydraulic\"}],\"Right\":[{\"id\":\"B\",\"label\":\"B\",\"type\":\"foundation.hydraulic.hydraulic\"}],\"Top\":[]}"
  Hydraulic Flow Rate Sensor : fl_lib/Hydraulic/Hydraulic Sensors/Hydraulic Flow Rate Sensor
  Hydraulic Flow Rate Source : fl_lib/Hydraulic/Hydraulic Sources/Hydraulic Flow Rate Source
      settings: InternalSimscapePortConfiguration="{\"Bottom\":[],\"Left\":[{\"id\":\"P\",\"label\":\"P\",\"type\":\"foundation.hydraulic.hydraulic\"}],\"Right\":[{\"id\":\"S\",\"label\":\"S\",\"type\":\"input\"},{\"id\":\"T\",\"label\":\"T\",\"type\":\"foundation.hydraulic.hydraulic\"}],\"Top\":[]}"
  Hydraulic Pressure Sensor : fl_lib/Hydraulic/Hydraulic Sensors/Hydraulic Pressure Sensor
  Hydraulic Pressure Source2 : fl_lib/Hydraulic/Hydraulic Sources/Hydraulic Pressure Source
      settings: InternalSimscapePortConfiguration="{\"Bottom\":[],\"Left\":[{\"id\":\"P\",\"label\":\"P\",\"type\":\"foundation.hydraulic.hydraulic\"}],\"Right\":[{\"id\":\"S\",\"label\":\"S\",\"type\":\"input\"},{\"id\":\"T\",\"label\":\"T\",\"type\":\"foundation.hydraulic.hydraulic\"}],\"Top\":[]}"
  Hydraulic Reference : fl_lib/Hydraulic/Hydraulic Elements/Hydraulic Reference
  PS Saturation : fl_lib/Physical Signals/Nonlinear Operators/PS Saturation  upper_limit=inf m^3/s  lower_limit=0 m^3/s
  PS Saturation1 : fl_lib/Physical Signals/Nonlinear Operators/PS Saturation  upper_limit=inf Pa  lower_limit=0 Pa
  PS Transfer Function : fl_lib/Physical Signals/Linear Operators/PS Transfer Function  transfer_function_type=foundation.enum.transfer_function_type.lag  T=tsample s  T1=2 s  T2=1 s  reset_method=foundation.enum.IntegratorResetSpec.None  initial_condition_spec=foundation.enum.IntegratorICSpec.Internal  y0=0 m^3/s
      settings: InternalSimscapePortConfiguration="{\"Bottom\":[],\"Left\":[{\"id\":\"U\",\"label\":\"\",\"type\":\"input\"}],\"Right\":[{\"id\":\"Y\",\"label\":\"\",\"type\":\"output\"}],\"Top\":[]}"
  PS Transfer Function1 : fl_lib/Physical Signals/Linear Operators/PS Transfer Function  transfer_function_type=foundation.enum.transfer_function_type.lag  T=tsample s  T1=2 s  T2=1 s  reset_method=foundation.enum.IntegratorResetSpec.None  initial_condition_spec=foundation.enum.IntegratorICSpec.Internal  y0=0 Pa
      settings: InternalSimscapePortConfiguration="{\"Bottom\":[],\"Left\":[{\"id\":\"U\",\"label\":\"\",\"type\":\"input\"}],\"Right\":[{\"id\":\"Y\",\"label\":\"\",\"type\":\"output\"}],\"Top\":[]}"
  A : PMIOPort  Side=Left
  B : PMIOPort  Port=2  Side=Right
  connections:
  Hydraulic Flow Rate Sensor/RConn2 -- Constant Area Hydraulic Orifice6/LConn1
  Constant Area Hydraulic Orifice6/RConn1 -- Hydraulic Reference/LConn1 -- Hydraulic Pressure Source2/RConn2
  Hydraulic Pressure Source2/LConn1 -- Hydraulic Flow Rate Sensor/LConn1
  Hydraulic Flow Rate Source/LConn1 -- Hydraulic Pressure Sensor/RConn1 -- Constant Area Hydraulic Orifice5/RConn1 -- B/RConn1
  PS Saturation/LConn1 -- Hydraulic Flow Rate Sensor/RConn1
  PS Transfer Function1/RConn1 -- Hydraulic Pressure Source2/RConn1
  Hydraulic Pressure Sensor/RConn2 -- PS Saturation1/LConn1
  Hydraulic Flow Rate Source/RConn2 -- Hydraulic Pressure Sensor/LConn1 -- A/RConn1 -- Constant Area Hydraulic Orifice5/LConn1
  PS Transfer Function/RConn1 -- Hydraulic Flow Rate Source/RConn1
  PS Saturation1/RConn1 -- PS Transfer Function1/LConn1
  PS Transfer Function/LConn1 -- PS Saturation/RConn1

== system hdv_hydroelectropowertrain_model/PR776_powertrain/Hydrostatic_powertrain/driveline_RD2/vd_ctrl_motor_RD/hose3 ==
  Constant Area Hydraulic Orifice : fl_lib/Hydraulic/Hydraulic Elements/Constant Area Hydraulic Orifice  area=1e-8 m^2  C_d=0.7  lam_spec=1  B_lam=0.999  Re_cr=12  q_specify=off  q_priority=None  q=0.001 m^3/s  q_nominal_specify=off  q_nominal_unit=m^3/s  q_nominal_value=1  p_specify=off  p_priority=None  p=0 Pa  p_nominal_specify=off  p_nominal_unit=Pa  p_nominal_value=1
      settings: InternalSimscapePortConfiguration="{\"Bottom\":[],\"Left\":[{\"id\":\"A\",\"label\":\"A\",\"type\":\"foundation.hydraulic.hydraulic\"}],\"Right\":[{\"id\":\"B\",\"label\":\"B\",\"type\":\"foundation.hydraulic.hydraulic\"}],\"Top\":[]}"
  Constant Area Hydraulic Orifice1 : fl_lib/Hydraulic/Hydraulic Elements/Constant Area Hydraulic Orifice  area=1e-8 m^2  C_d=0.7  lam_spec=1  B_lam=0.999  Re_cr=12  q_specify=off  q_priority=None  q=0.001 m^3/s  q_nominal_specify=off  q_nominal_unit=m^3/s  q_nominal_value=1  p_specify=off  p_priority=None  p=0 Pa  p_nominal_specify=off  p_nominal_unit=Pa  p_nominal_value=1
      settings: InternalSimscapePortConfiguration="{\"Bottom\":[],\"Left\":[{\"id\":\"A\",\"label\":\"A\",\"type\":\"foundation.hydraulic.hydraulic\"}],\"Right\":[{\"id\":\"B\",\"label\":\"B\",\"type\":\"foundation.hydraulic.hydraulic\"}],\"Top\":[]}"
  Hydraulic Flow Rate Sensor3 : fl_lib/Hydraulic/Hydraulic Sensors/Hydraulic Flow Rate Sensor
  Hydraulic Flow Rate Source : fl_lib/Hydraulic/Hydraulic Sources/Hydraulic Flow Rate Source
      settings: InternalSimscapePortConfiguration="{\"Bottom\":[],\"Left\":[{\"id\":\"P\",\"label\":\"P\",\"type\":\"foundation.hydraulic.hydraulic\"}],\"Right\":[{\"id\":\"S\",\"label\":\"S\",\"type\":\"input\"},{\"id\":\"T\",\"label\":\"T\",\"type\":\"foundation.hydraulic.hydraulic\"}],\"Top\":[]}"
  Hydraulic Pressure Sensor2 : fl_lib/Hydraulic/Hydraulic Sensors/Hydraulic Pressure Sensor
  Hydraulic Pressure Source : fl_lib/Hydraulic/Hydraulic Sources/Hydraulic Pressure Source
      settings: InternalSimscapePortConfiguration="{\"Bottom\":[],\"Left\":[{\"id\":\"P\",\"label\":\"P\",\"type\":\"foundation.hydraulic.hydraulic\"}],\"Right\":[{\"id\":\"S\",\"label\":\"S\",\"type\":\"input\"},{\"id\":\"T\",\"label\":\"T\",\"type\":\"foundation.hydraulic.hydraulic\"}],\"Top\":[]}"
  Hydraulic Reference : fl_lib/Hydraulic/Hydraulic Elements/Hydraulic Reference
  PS Gain : fl_lib/Physical Signals/Functions/PS Gain  gain=1 Pa
  PS Gain1 : fl_lib/Physical Signals/Functions/PS Gain  gain=1 Pa^-1
  PS Gain2 : fl_lib/Physical Signals/Functions/PS Gain  gain=1 m^3/s
  PS Gain3 : fl_lib/Physical Signals/Functions/PS Gain  gain=1 m^-3*s
  PS Transfer Function : fl_lib/Physical Signals/Linear Operators/PS Transfer Function  transfer_function_type=foundation.enum.transfer_function_type.lag  T=0.01 s  T1=2 s  T2=1 s  reset_method=foundation.enum.IntegratorResetSpec.None  initial_condition_spec=foundation.enum.IntegratorICSpec.Internal  y0=0
      settings: InternalSimscapePortConfiguration="{\"Bottom\":[],\"Left\":[{\"id\":\"U\",\"label\":\"\",\"type\":\"input\"}],\"Right\":[{\"id\":\"Y\",\"label\":\"\",\"type\":\"output\"}],\"Top\":[]}"
  PS Transfer Function1 : fl_lib/Physical Signals/Linear Operators/PS Transfer Function  transfer_function_type=foundation.enum.transfer_function_type.lag  T=0.01 s  T1=2 s  T2=1 s  reset_method=foundation.enum.IntegratorResetSpec.None  initial_condition_spec=foundation.enum.IntegratorICSpec.Internal  y0=0
      settings: InternalSimscapePortConfiguration="{\"Bottom\":[],\"Left\":[{\"id\":\"U\",\"label\":\"\",\"type\":\"input\"}],\"Right\":[{\"id\":\"Y\",\"label\":\"\",\"type\":\"output\"}],\"Top\":[]}"
  A : PMIOPort  Side=Left
  AA : PMIOPort  Port=2  Side=Right
  B : PMIOPort  Port=3  Side=Left
  BB : PMIOPort  Port=4  Side=Right
  connections:
  PS Gain1/RConn1 -- PS Transfer Function/LConn1
  PS Gain3/RConn1 -- PS Transfer Function1/LConn1
  Hydraulic Flow Rate Source/RConn2 -- Hydraulic Pressure Sensor2/LConn1 -- Constant Area Hydraulic Orifice/LConn1 -- A/RConn1
  PS Transfer Function/RConn1 -- PS Gain/LConn1
  PS Transfer Function1/RConn1 -- PS Gain2/LConn1
  BB/RConn1 -- Hydraulic Reference/LConn1 -- Constant Area Hydraulic Orifice1/RConn1 -- Hydraulic Flow Rate Source/LConn1 -- B/RConn1 -- Constant Area Hydraulic Orifice/RConn1 -- Hydraulic Pressure Sensor2/RConn1 -- Hydraulic Pressure Source/RConn2
  PS Gain1/LConn1 -- Hydraulic Pressure Sensor2/RConn2
  Hydraulic Pressure Source/RConn1 -- PS Gain/RConn1
  Hydraulic Flow Rate Sensor3/LConn1 -- Hydraulic Pressure Source/LConn1
  Hydraulic Flow Rate Sensor3/RConn1 -- PS Gain3/LConn1
  PS Gain2/RConn1 -- Hydraulic Flow Rate Source/RConn1
  Hydraulic Flow Rate Sensor3/RConn2 -- Constant Area Hydraulic Orifice1/LConn1 -- AA/RConn1

== system hdv_hydroelectropowertrain_model/PR776_powertrain/Hydrostatic_powertrain/driveline_RD2/vd_ctrl_motor_RD/servo motor LD ==
  displacement reference pu : Inport
  PS Add : fl_lib/Physical Signals/Functions/PS Add
  PS Constant : fl_lib/Physical Signals/Sources/PS Constant  constant=1
  PS Gain : fl_lib/Physical Signals/Functions/PS Gain  gain=-1/0.06 m^-1
  hydrostatic_threeway_valve_bichamber_piston : hydrostatic_threeway_valve_bichamber_piston_lib/hydrostatic_threeway_valve_bichamber_piston  Dh=Dh m  Dr=Dr m  Lp=Lpm m  xv_max=xv_m_max mm  mp=mp_m kg  kp=kp_m N/m  bp=bp_m N/(m/s)  qs_specify=off  qs_priority=None  qs=0 m^3/s  qs_nominal_specify=off  qs_nominal_unit=m^3/s  qs_nominal_value=1  qv_specify=off  qv_priority=None  qv=0 m^3/s  qv_nominal_specify=off  qv_nominal_unit=m^3/s  qv_nominal_value=1  q_specify=off  q_priority=None  q=0 m^3/s  q_nominal_specify=off  q_nominal_unit=m^3/s  q_nominal_value=1  q_leak_specify=off  q_leak_priority=None  q_leak=0 m^3/s  q_leak_nominal_specify=off  q_leak_nominal_unit=m^3/s  q_leak_nominal_value=1  pc_specify=off  pc_priority=None  pc=0 bar  pc_nominal_specify=off  pc_nominal_unit=bar  pc_nominal_value=1  fp_specify=off  fp_priority=None  fp=0 N  fp_nominal_specify=off  fp_nominal_unit=N  fp_nominal_value=1  vp_specify=off  vp_priority=None  vp=0 m/s  vp_nominal_specify=off  vp_nominal_unit=m/s  vp_nominal_value=1  xp_specify=off  xp_priority=High  xp=10 mm  xp_nominal_specify=off  xp_nominal_unit=mm  xp_nominal_value=1
      settings: InternalSimscapePortConfiguration="{\"Bottom\":[],\"Left\":[{\"id\":\"xv\",\"label\":\"xv\",\"type\":\"input\"},{\"id\":\"cA\",\"label\":\"cA\",\"type\":\"foundation.hydraulic.hydraulic\"},{\"id\":\"cB\",\"label\":\"cB\",\"type\":\"foundation.hydraulic.hydraulic\"}],\"Right\":[{\"id\":\"P\",\"label\":\"P\",\"type\":\"foundation.mechanical.translational.translational\"},{\"id\":\"xp_out\",\"label\":\"xp\",\"type\":\"output\"},{\"id\":\"mforce\",\"label\":\"fm\",\"type\":\"output\"},{\"id\":\"flowC\",\"label\":\"flowC\",\"type\":\"output\"},{\"id\":\"pC\",\"label\":\"pC\",\"type\":\"output\"}],\"Top\":[]}"
  servo_ctrl : Subsystem
  pS : PMIOPort  Side=Left
  pT : PMIOPort  Port=2  Side=Left
  vd : PMIOPort  Port=3  Side=Right
  wires:
  displacement reference pu/1 -> servo_ctrl/1(ref)
  connections:
  PS Constant/RConn1 -- PS Add/LConn2
  PS Gain/RConn1 -- PS Add/LConn1
  vd/RConn1 -- PS Add/RConn1
  hydrostatic_threeway_valve_bichamber_piston/LConn1 -- servo_ctrl/RConn1
  servo_ctrl/LConn1 -- PS Gain/LConn1 -- hydrostatic_threeway_valve_bichamber_piston/RConn2
  hydrostatic_threeway_valve_bichamber_piston/LConn2 -- pS/RConn1
  hydrostatic_threeway_valve_bichamber_piston/LConn3 -- pT/RConn1

== system hdv_hydroelectropowertrain_model/PR776_powertrain/Hydrostatic_powertrain/driveline_RD2/vd_ctrl_pump_RD/hose3 ==
  Constant Area Hydraulic Orifice : fl_lib/Hydraulic/Hydraulic Elements/Constant Area Hydraulic Orifice  area=1e-8 m^2  C_d=0.7  lam_spec=1  B_lam=0.999  Re_cr=12  q_specify=off  q_priority=None  q=0.001 m^3/s  q_nominal_specify=off  q_nominal_unit=m^3/s  q_nominal_value=1  p_specify=off  p_priority=None  p=0 Pa  p_nominal_specify=off  p_nominal_unit=Pa  p_nominal_value=1
      settings: InternalSimscapePortConfiguration="{\"Bottom\":[],\"Left\":[{\"id\":\"A\",\"label\":\"A\",\"type\":\"foundation.hydraulic.hydraulic\"}],\"Right\":[{\"id\":\"B\",\"label\":\"B\",\"type\":\"foundation.hydraulic.hydraulic\"}],\"Top\":[]}"
  Constant Area Hydraulic Orifice1 : fl_lib/Hydraulic/Hydraulic Elements/Constant Area Hydraulic Orifice  area=1e-8 m^2  C_d=0.7  lam_spec=1  B_lam=0.999  Re_cr=12  q_specify=off  q_priority=None  q=0.001 m^3/s  q_nominal_specify=off  q_nominal_unit=m^3/s  q_nominal_value=1  p_specify=off  p_priority=None  p=0 Pa  p_nominal_specify=off  p_nominal_unit=Pa  p_nominal_value=1
      settings: InternalSimscapePortConfiguration="{\"Bottom\":[],\"Left\":[{\"id\":\"A\",\"label\":\"A\",\"type\":\"foundation.hydraulic.hydraulic\"}],\"Right\":[{\"id\":\"B\",\"label\":\"B\",\"type\":\"foundation.hydraulic.hydraulic\"}],\"Top\":[]}"
  Hydraulic Flow Rate Sensor3 : fl_lib/Hydraulic/Hydraulic Sensors/Hydraulic Flow Rate Sensor
  Hydraulic Flow Rate Source : fl_lib/Hydraulic/Hydraulic Sources/Hydraulic Flow Rate Source
      settings: InternalSimscapePortConfiguration="{\"Bottom\":[],\"Left\":[{\"id\":\"P\",\"label\":\"P\",\"type\":\"foundation.hydraulic.hydraulic\"}],\"Right\":[{\"id\":\"S\",\"label\":\"S\",\"type\":\"input\"},{\"id\":\"T\",\"label\":\"T\",\"type\":\"foundation.hydraulic.hydraulic\"}],\"Top\":[]}"
  Hydraulic Pressure Sensor2 : fl_lib/Hydraulic/Hydraulic Sensors/Hydraulic Pressure Sensor
  Hydraulic Pressure Source : fl_lib/Hydraulic/Hydraulic Sources/Hydraulic Pressure Source
      settings: InternalSimscapePortConfiguration="{\"Bottom\":[],\"Left\":[{\"id\":\"P\",\"label\":\"P\",\"type\":\"foundation.hydraulic.hydraulic\"}],\"Right\":[{\"id\":\"S\",\"label\":\"S\",\"type\":\"input\"},{\"id\":\"T\",\"label\":\"T\",\"type\":\"foundation.hydraulic.hydraulic\"}],\"Top\":[]}"
  Hydraulic Reference : fl_lib/Hydraulic/Hydraulic Elements/Hydraulic Reference
  PS Gain : fl_lib/Physical Signals/Functions/PS Gain  gain=1 Pa
  PS Gain1 : fl_lib/Physical Signals/Functions/PS Gain  gain=1 Pa^-1
  PS Gain2 : fl_lib/Physical Signals/Functions/PS Gain  gain=1 m^3/s
  PS Gain3 : fl_lib/Physical Signals/Functions/PS Gain  gain=1 m^-3*s
  PS Transfer Function : fl_lib/Physical Signals/Linear Operators/PS Transfer Function  transfer_function_type=foundation.enum.transfer_function_type.lag  T=0.01 s  T1=2 s  T2=1 s  reset_method=foundation.enum.IntegratorResetSpec.None  initial_condition_spec=foundation.enum.IntegratorICSpec.Internal  y0=0
      settings: InternalSimscapePortConfiguration="{\"Bottom\":[],\"Left\":[{\"id\":\"U\",\"label\":\"\",\"type\":\"input\"}],\"Right\":[{\"id\":\"Y\",\"label\":\"\",\"type\":\"output\"}],\"Top\":[]}"
  PS Transfer Function1 : fl_lib/Physical Signals/Linear Operators/PS Transfer Function  transfer_function_type=foundation.enum.transfer_function_type.lag  T=0.01 s  T1=2 s  T2=1 s  reset_method=foundation.enum.IntegratorResetSpec.None  initial_condition_spec=foundation.enum.IntegratorICSpec.Internal  y0=0
      settings: InternalSimscapePortConfiguration="{\"Bottom\":[],\"Left\":[{\"id\":\"U\",\"label\":\"\",\"type\":\"input\"}],\"Right\":[{\"id\":\"Y\",\"label\":\"\",\"type\":\"output\"}],\"Top\":[]}"
  A : PMIOPort  Side=Left
  AA : PMIOPort  Port=2  Side=Right
  B : PMIOPort  Port=3  Side=Left
  BB : PMIOPort  Port=4  Side=Right
  connections:
  PS Gain1/RConn1 -- PS Transfer Function/LConn1
  PS Gain3/RConn1 -- PS Transfer Function1/LConn1
  Hydraulic Flow Rate Source/RConn2 -- Hydraulic Pressure Sensor2/LConn1 -- Constant Area Hydraulic Orifice/LConn1 -- A/RConn1
  PS Transfer Function/RConn1 -- PS Gain/LConn1
  PS Transfer Function1/RConn1 -- PS Gain2/LConn1
  BB/RConn1 -- Hydraulic Reference/LConn1 -- Constant Area Hydraulic Orifice1/RConn1 -- Hydraulic Flow Rate Source/LConn1 -- B/RConn1 -- Constant Area Hydraulic Orifice/RConn1 -- Hydraulic Pressure Sensor2/RConn1 -- Hydraulic Pressure Source/RConn2
  PS Gain1/LConn1 -- Hydraulic Pressure Sensor2/RConn2
  Hydraulic Pressure Source/RConn1 -- PS Gain/RConn1
  Hydraulic Flow Rate Sensor3/LConn1 -- Hydraulic Pressure Source/LConn1
  Hydraulic Flow Rate Sensor3/RConn1 -- PS Gain3/LConn1
  PS Gain2/RConn1 -- Hydraulic Flow Rate Source/RConn1
  Hydraulic Flow Rate Sensor3/RConn2 -- Constant Area Hydraulic Orifice1/LConn1 -- AA/RConn1
